simulink model "untitled"  (R2021a)
settings: Solver=FixedStepAuto  StartTime=0.0  StopTime=20  FixedStep=.05  RelTol=1e-3
InitFcn:
  | parameters
values from neighbouring files (symbols this model uses):
  e3 = [0 0 1]'    [parameters.m]
  g = 9.81    [parameters.m]
  J = diag([0.0820; 0.0845; 0.1377])    [parameters.m]
  m = 4.34    [parameters.m]
  omega_0 = [0 0 0]'    [parameters.m]
  R_0 = eye(3)    [parameters.m]
  rotor_matrix = [1 1 1 1;0 -d 0 d;d 0 -d 0;-ctauf ctauf -ctauf ctauf]    [parameters.m]
  v_0 = [0 0 0]'    [parameters.m]
  x_0 = [0 0 0]'    [parameters.m]
libraries: vrlib x1
settings Model: Creator=hamed.habibi  LastModifiedBy=hamed.habibi
settings DataIOCC: ReturnWorkspaceOutputs=off

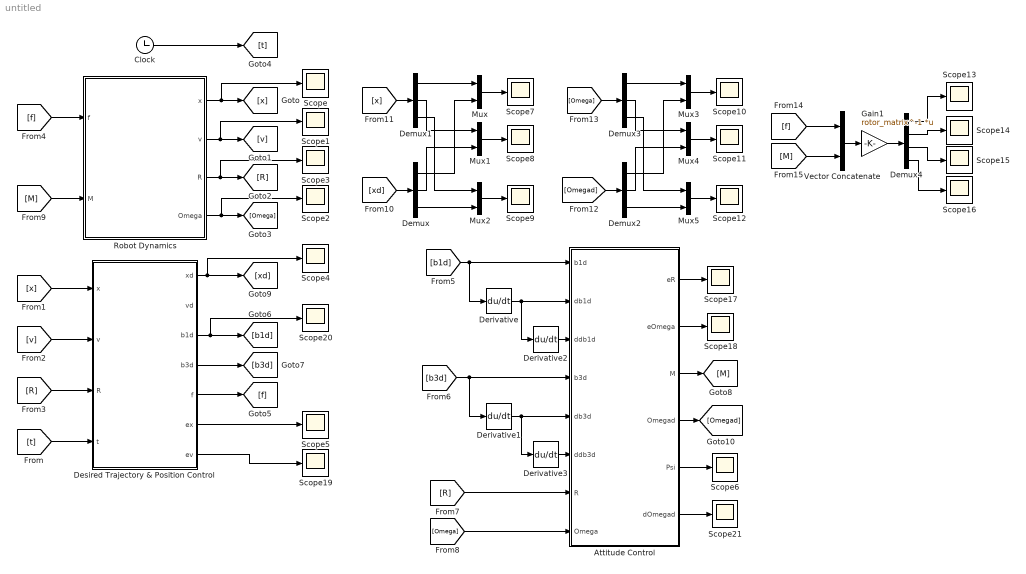
== system untitled ==
  Attitude Control : MATLAB Function  TreatAsAtomicUnit=on
  Clock : Clock
  Demux{,1..3} (4 alike) : Demux  Outputs=3
  Demux4 : Demux
  Derivative{,1..3} (4 alike) : Derivative
  Desired Trajectory & Position Control : MATLAB Function  TreatAsAtomicUnit=on
  Gain1 : Gain  Gain=rotor_matrix^-1  Multiplication=Matrix(K*u)
  Mux{,1..5} (6 alike) : Mux  Inputs=2
  Robot Dynamics : Subsystem
  Scope{,1..21} (22 alike) : Scope
  Vector Concatenate : Concatenate
  wires:
  [f] -> Robot Dynamics/1(f)
  [M] -> Robot Dynamics/2(M)
  Robot Dynamics/1(x) -> [x], Scope/1
  Robot Dynamics/2(v) -> Scope1/1, [v]
  Robot Dynamics/3(R) -> Scope3/1, [R]
  Robot Dynamics/4(Omega) -> [Omega], Scope2/1
  Clock/1 -> [t]
  [v] -> Desired Trajectory & Position Control/2(v)
  [x] -> Desired Trajectory & Position Control/1(x)
  [t] -> Desired Trajectory & Position Control/4(t)
  [R] -> Desired Trajectory & Position Control/3(R)
  Desired Trajectory & Position Control/5(f) -> [f]
  Desired Trajectory & Position Control/1(xd) -> [xd], Scope4/1
  Desired Trajectory & Position Control/6(ex) -> Scope5/1
  Desired Trajectory & Position Control/4(b3d) -> [b3d]
  Desired Trajectory & Position Control/3(b1d) -> Scope20/1, [b1d]
  [b1d] -> Attitude Control/1(b1d), Derivative/1
  [b3d] -> Derivative1/1, Attitude Control/4(b3d)
  Derivative/1 -> Derivative2/1, Attitude Control/2(db1d)
  Derivative1/1 -> Attitude Control/5(db3d), Derivative3/1
  [R] -> Attitude Control/7(R)
  [Omega] -> Attitude Control/8(Omega)
  Attitude Control/3(M) -> [M]
  Attitude Control/5(Psi) -> Scope6/1
  [xd] -> Demux/1
  [x] -> Demux1/1
  Mux/1 -> Scope7/1
  Mux1/1 -> Scope8/1
  Mux2/1 -> Scope9/1
  Demux1/1 -> Mux/1
  Demux/1 -> Mux/2
  Demux1/2 -> Mux1/1
  Demux/2 -> Mux1/2
  Demux1/3 -> Mux2/1
  Demux/3 -> Mux2/2
  Demux2/3 -> Mux5/2
  Demux3/3 -> Mux5/1
  Demux2/2 -> Mux4/2
  Demux3/2 -> Mux4/1
  Demux2/1 -> Mux3/2
  Demux3/1 -> Mux3/1
  Mux5/1 -> Scope12/1
  Mux4/1 -> Scope11/1
  Mux3/1 -> Scope10/1
  [Omega] -> Demux3/1
  [Omegad] -> Demux2/1
  Attitude Control/4(Omegad) -> [Omegad]
  [M] -> Vector Concatenate/2
  [f] -> Vector Concatenate/1
  Vector Concatenate/1 -> Gain1/1
  Gain1/1 -> Demux4/1
  Demux4/1 -> Scope13/1
  Demux4/2 -> Scope14/1
  Demux4/3 -> Scope15/1
  Demux4/4 -> Scope16/1
  Attitude Control/1(eR) -> Scope17/1
  Attitude Control/2(eOmega) -> Scope18/1
  Desired Trajectory & Position Control/7(ev) -> Scope19/1
  Derivative2/1 -> Attitude Control/3(ddb1d)
  Derivative3/1 -> Attitude Control/6(ddb3d)
  Attitude Control/6(dOmegad) -> Scope21/1

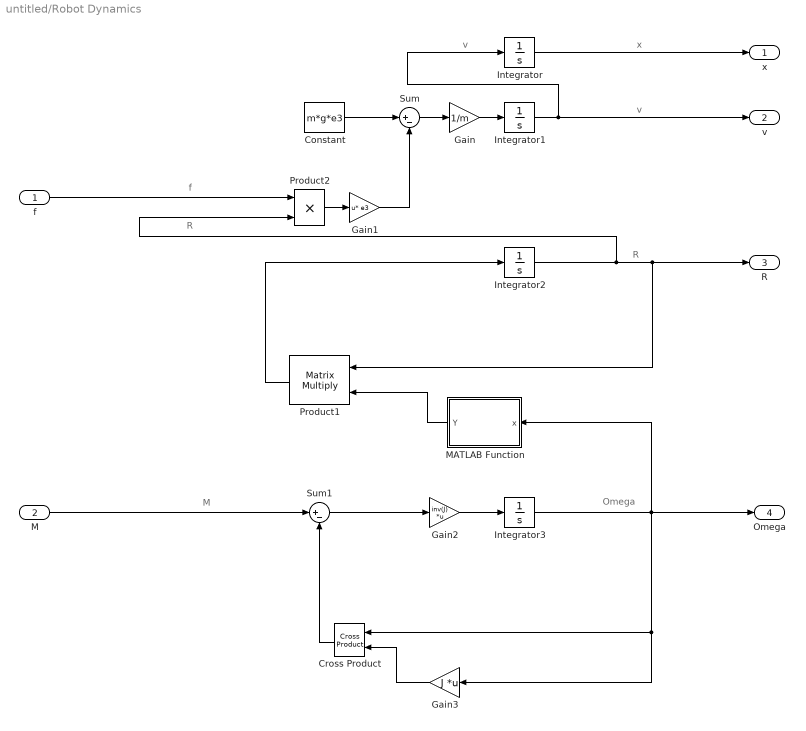
== system untitled/Robot Dynamics ==
  note: M
  note: R
  note: R
  note: f
  note: v
  note: v
  note: Omega
  note: x
  f : Inport
  M : Inport  Port=2
  Constant : Constant  Value=m*g*e3
  Cross Product : vrlib/Utilities/Cross Product
  Gain : Gain  Gain=1/m
  Gain1 : Gain  Gain=e3  Multiplication=Matrix(u*K)
  Gain2 : Gain  Gain=inv(J)  Multiplication=Matrix(K*u) (u vector)
  Gain3 : Gain  Gain=J  Multiplication=Matrix(K*u) (u vector)
  Integrator : Integrator  InitialCondition=x_0
  Integrator1 : Integrator  InitialCondition=v_0
  Integrator2 : Integrator  InitialCondition=R_0
  Integrator3 : Integrator  InitialCondition=omega_0
  MATLAB Function : MATLAB Function  TreatAsAtomicUnit=on
  Product1 : Product  Multiplication=Matrix(*)
  Product2 : Product
  Sum : Sum  Inputs=|+-
  Sum1 : Sum  Inputs=|+-
  x : Outport
  v : Outport  Port=2
  R : Outport  Port=3
  Omega : Outport  Port=4
  wires:
  Integrator1/1 -> v/1, Integrator/1
  Product2/1 -> Gain1/1
  Integrator/1 -> x/1
  Gain1/1 -> Sum/2
  Integrator3/1 -> Omega/1, Cross Product/1, Gain3/1, MATLAB Function/1(x)
  Sum/1 -> Gain/1
  f/1 -> Product2/1
  Integrator2/1 -> Product2/2, R/1, Product1/1
  Product1/1 -> Integrator2/1
  MATLAB Function/1(Y) -> Product1/2
  Cross Product/1 -> Sum1/2
  Gain2/1 -> Integrator3/1
  Gain3/1 -> Cross Product/2
  Sum1/1 -> Gain2/1
  Gain/1 -> Integrator1/1
  Constant/1 -> Sum/1
  M/1 -> Sum1/1

== matlab function untitled/Desired Trajectory & Position Control ==
  data: x input; v input; R input; t input; xd output; vd output; b1d output; b3d output; f output; ex output; ev output
function [xd,vd,b1d,b3d,f,ex,ev]= fcn(x, v, R, t)
m = 4.34;
kx = 16;
kv = 5.6;
e3 = [0 0 1]';
g = 9.81;
xd = [.4*t .4*sin(pi*t) .6*cos(pi*t)]';
vd = [.4 .4*pi*cos(pi*t) -.6*pi*sin(pi*t)]';
ddxd = [0 -.4*pi*pi*sin(pi*t) -.6*pi*pi*cos(pi*t)]';
b1d = [cos(pi*t) sin(pi*t) 0]';
ex = x-xd;
ev = v-vd;
num = -kx*ex-kv*ev-m*g*e3+m*ddxd;
den = norm(num);
b3d = num/den;
f=-num'*R*e3;

== matlab function untitled/Robot Dynamics/MATLAB Function ==
  data: x input; Y output
function Y=skew(x)
Y=[0 -x(3) x(2) ; x(3) 0 -x(1) ; -x(2) x(1) 0 ];

== matlab function untitled/Attitude Control ==
  data: b1d input; db1d input; ddb1d input; eR output; b3d input; db3d input; ddb3d input; R input; Omega input; eOmega output; M output; Omegad output; Psi output; dOmegad output
function [eR,eOmega,M,Omegad,Psi,dOmegad] = fcn(b1d,db1d,ddb1d,b3d,db3d,ddb3d,R,Omega)
kR = 8.81;
kOmega = 2.54;
J = diag([0.0820; 0.0845; 0.1377]);
num=cross(b3d,b1d);
den=norm(num);
dnum=cross(db3d,b1d)+cross(b3d,db1d);
dden=(dnum'*num+num'*dnum)/2/sqrt(num'*num);
b2d=num/den;
db2d=(dnum*den-num*dden)/(den^2);
Rd=[cross(b2d,b3d),b2d,b3d];
term=cross(db2d,b3d)+cross(b2d,db3d);
dRd=[term,db2d,db3d];
X=.5*(Rd'*R-R'*Rd);
eR=[-X(2,3);X(1,3);-X(1,2)];
Y=Rd'*dRd;
Omegad=[-Y(2,3);Y(1,3);-Y(1,2)];
%
ddnum=cross(ddb3d,b1d)+cross(db3d,db1d)+cross(db3d,db1d)+cross(b3d,ddb1d);
ddden=(2*norm(num)*(ddnum'*num+dnum'*dnum+dnum'*dnum+num'*ddnum)-2*(dnum'*num+num'*dnum)*dden)/4/norm(num)^2;
ddb2d=(den^2*(ddnum*den-num*ddden)-2*dden*den*(dnum*den-num*dden))/den^4;
dterm=cross(ddb2d,b3d)+cross(db2d,db3d)+cross(db2d,db3d)+cross(b2d,ddb3d);
ddRd=[dterm,ddb2d,ddb3d];
W=dRd'*dRd+Rd'*ddRd;
dOmegad=[-W(2,3);W(1,3);-W(1,2)];
%
%dOmegad=.01*[1 1 1]';
eOmega=Omega-R'*Rd*Omegad;
OmegaSkew=[0 -Omega(3) Omega(2) ; Omega(3) 0 -Omega(1) ; -Omega(2) Omega(1) 0 ];
M=-kR*eR-kOmega*eOmega+cross(Omega,J*Omega)-J*(OmegaSkew*R'*Rd*Omegad-R'*Rd*dOmegad);
Psi=.5*trace(eye(3)-Rd'*R);
